simulink model "Simulation_2020b"  (R2020b)
settings: Solver=VariableStepAuto  StartTime=0.0  StopTime=15  RelTol=1e-3
undefined symbols (not defined in the file): A, B, C, D, data, National_Instruments, PCIe
libraries: sldrtlib x2, SignalEditorBlockLib x1
settings Model: Creator=ematric  LastModifiedBy=EAL
settings DebuggingCC: UnconnectedInputMsg=none  UnconnectedOutputMsg=none  UnconnectedLineMsg=none
settings ModelReferenceCC: EnableRefExpFcnMdlSchedulingChecks=off

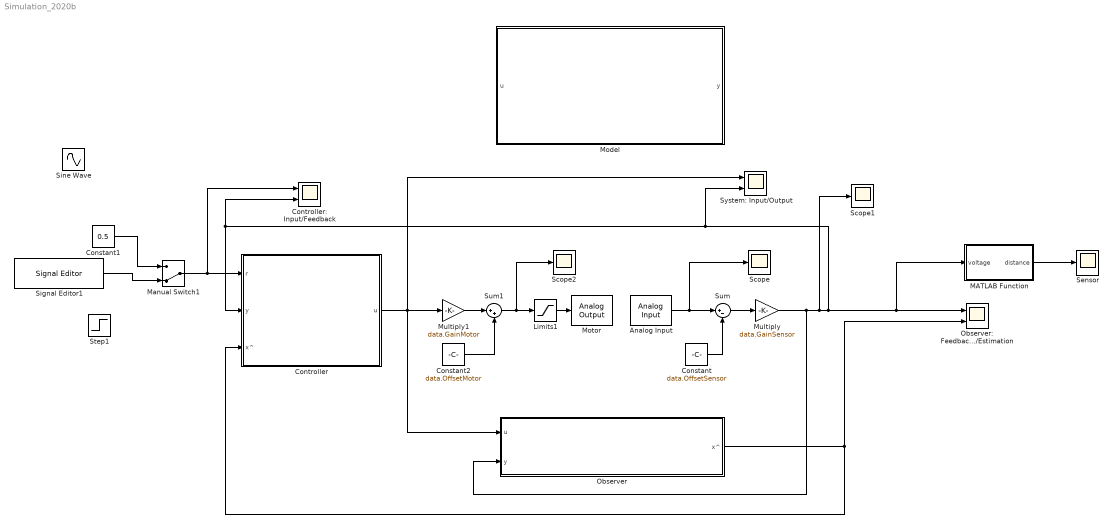
== system Simulation_2020b ==
  Analog Input : sldrtlib/Analog Input  SampleTime=0.1  MaxMissedTicks=10  ShowMissedTicks=off  YieldWhenWaiting=off  DrvName=National_Instruments/PCIe-6321  DrvAddress=4294967295  DrvOptions=[0 0 0 0 0 0 0]  Channels=1  RangeMode=1  VoltRange=1  DataType=1
      settings: AttributesFormatString=National Instruments\nPCIe-6321 [auto]
  Constant : Constant  Value=data.OffsetSensor
  Constant1 : Constant  Value=0.5
  Constant2 : Constant  Value=data.OffsetMotor
  Controller : Subsystem
  Controller: Input/Feedback : Scope  NumInputPorts=2
  Limits1 : Saturate  UpperLimit=5  LowerLimit=-5
  MATLAB Function : MATLAB Function  TreatAsAtomicUnit=on
  Manual Switch1 : ManualSwitch  CurrentSetting=0
  Model : Subsystem
  Motor : sldrtlib/Analog Output  SampleTime=0.1  MaxMissedTicks=10  ShowMissedTicks=off  YieldWhenWaiting=off  DrvName=National_Instruments/PCIe-6321  DrvAddress=4294967295  DrvOptions=[0 0 0 0 0 0 0]  Channels=1  RangeMode=1  VoltRange=1  InitialValue=0  FinalValue=0
      settings: AttributesFormatString=National Instruments\nPCIe-6321 [auto]
  Multiply : Gain  Gain=data.GainSensor
  Multiply1 : Gain  Gain=data.GainMotor
  "Observer " : Subsystem
  Observer: Feedback/Estimation : Scope  NumInputPorts=2
  Scope : Scope
  Scope1 : Scope
  Scope2 : Scope
  Sensor : Scope
  Signal Editor1 : SignalEditorBlockLib/Signal Editor  FileName=C:\Users\EAL\Desktop\Preparation second lab (2B) Figl Sieß Widmann 2020\trajectories.mat  ActiveScenario=Scenario  ActiveSignal=TestSignal  IsBus=off  OutputBusObjectStr=Bus: BusObject  SampleTime=0  Interpolate=off  ZeroCross=off  OutputAfterFinalValue=Setting to zero  Unit=inherit  PreserveSignalName=on
  Sine Wave : Sin  Amplitude=0.5  Bias=0.5  Frequency=0.2  SampleTime=0
  Step1 : Step  After=0.5  SampleTime=0
  Sum : Sum  Inputs=|+-
  Sum1 : Sum  Inputs=|++
  System: Input/Output : Scope  NumInputPorts=2
  wires:
  "Observer "/1(x^) -> Controller/3(x^), Observer: Feedback/Estimation/2
  Manual Switch1/1 -> Controller: Input/Feedback/1, Controller/1(r)
  Sum/1 -> Multiply/1
  MATLAB Function/1(distance) -> Sensor/1
  Analog Input/1 -> Scope/1, Sum/1
  Constant/1 -> Sum/2
  Multiply/1 -> Scope1/1, MATLAB Function/1(voltage), Observer: Feedback/Estimation/1, System: Input/Output/2, Controller/2(y), Controller: Input/Feedback/2, "Observer "/2(y)
  Constant2/1 -> Sum1/2
  Controller/1(u) -> Multiply1/1, System: Input/Output/1, "Observer "/1(u)
  Multiply1/1 -> Sum1/1
  Sum1/1 -> Limits1/1, Scope2/1
  Limits1/1 -> Motor/1
  Signal Editor1/1 -> Manual Switch1/2
  Constant1/1 -> Manual Switch1/1

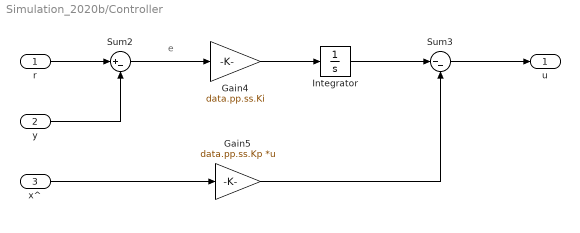
== system Simulation_2020b/Controller ==
  note: e
  r : Inport
  y : Inport  Port=2
  x^ : Inport  Port=3
  Gain4 : Gain  Gain=data.pp.ss.Ki
  Gain5 : Gain  Gain=data.pp.ss.Kp  Multiplication=Matrix(K*u)
  Integrator : Integrator
  Sum2 : Sum  Inputs=|+-
  Sum3 : Sum  Inputs=|--
  u : Outport
  wires:
  Integrator/1 -> Sum3/1
  Gain4/1 -> Integrator/1
  Sum2/1 -> Gain4/1
  Gain5/1 -> Sum3/2
  r/1 -> Sum2/1
  y/1 -> Sum2/2
  Sum3/1 -> u/1
  x^/1 -> Gain5/1

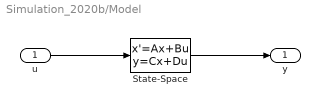
== system Simulation_2020b/Model ==
  u : Inport
  State-Space : StateSpace  A=A  B=B  C=C  D=D  InitialCondition=0
  y : Outport
  wires:
  u/1 -> State-Space/1
  State-Space/1 -> y/1

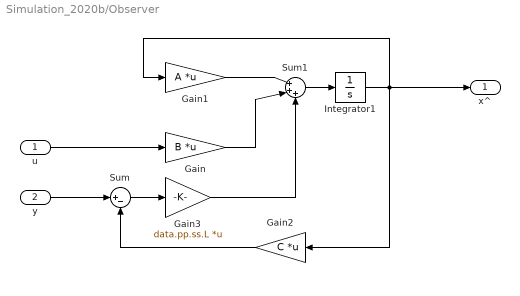
== system Simulation_2020b/Observer  ==
  u : Inport
  y : Inport  Port=2
  Gain : Gain  Gain=B  Multiplication=Matrix(K*u)
  Gain1 : Gain  Gain=A  Multiplication=Matrix(K*u)
  Gain2 : Gain  Gain=C  Multiplication=Matrix(K*u)
  Gain3 : Gain  Gain=data.pp.ss.L  Multiplication=Matrix(K*u)
  Integrator1 : Integrator
  Sum : Sum  Inputs=|+-
  Sum1 : Sum  Inputs=|+++
  x^ : Outport
  wires:
  Gain1/1 -> Sum1/1
  Gain2/1 -> Sum/2
  Sum/1 -> Gain3/1
  Integrator1/1 -> x^/1, Gain2/1, Gain1/1
  Gain/1 -> Sum1/2
  Gain3/1 -> Sum1/3
  Sum1/1 -> Integrator1/1
  u/1 -> Gain/1
  y/1 -> Sum/1

== matlab function Simulation_2020b/MATLAB Function ==
  data: voltage input; distance output
function distance = fcn(voltage)

distance=(73.3604*voltage.^3)+(-339.1311*voltage.^2)+(527.2338*voltage)+(-242.9424);
